simulink model "voertuig_cvs1"  (Simulink 8.0)
settings: Solver=ode45  StartTime=0.0  StopTime=simtijd  MaxStep=0.2  RelTol=1e-3
values from neighbouring files (symbols this model uses):
  Cw = 0.3    [voertuigmodel_rvv.m]
  fr = 0.014    [voertuigmodel_rvv.m]
  g = 9.81    [voertuigmodel_rvv.m]
  i = [1 2 3 4 5; 12 7.5 5.5 4.5 3.75]'    [voertuigmodel_rvv.m]
  J1 = 1.2    [voertuigmodel_rvv.m]
  J2 = 5.4    [voertuigmodel_rvv.m]
  m = 950    [voertuigmodel_rvv.m]
  mu_max = 1.05    [voertuigmodel_rvv.m]
  Nm_motor = [0 1000 2000 3000 4000 5000 6000 6500 7000; 50 90 90 95 100 90 85 80 0]'    [voertuigmodel_rvv.m]
  r = 0.3    [voertuigmodel_rvv.m]
  rho = 1.29    [voertuigmodel_rvv.m]
  v_i = [1 2 3 4 5;0 4.17 8.89 13.89 19.44]'    [voertuigmodel_rvv.m]
libraries: simulink x2
settings Model: Creator=879618  LastModifiedBy=879618
settings DataIOCC: SignalLoggingSaveFormat=ModelDataLogs
settings DebuggingCC: FcnCallInpInsideContextMsg=EnableAllAsWarning
settings GRTTargetCC: CombineOutputUpdateFcns=off  GRTInterface=on

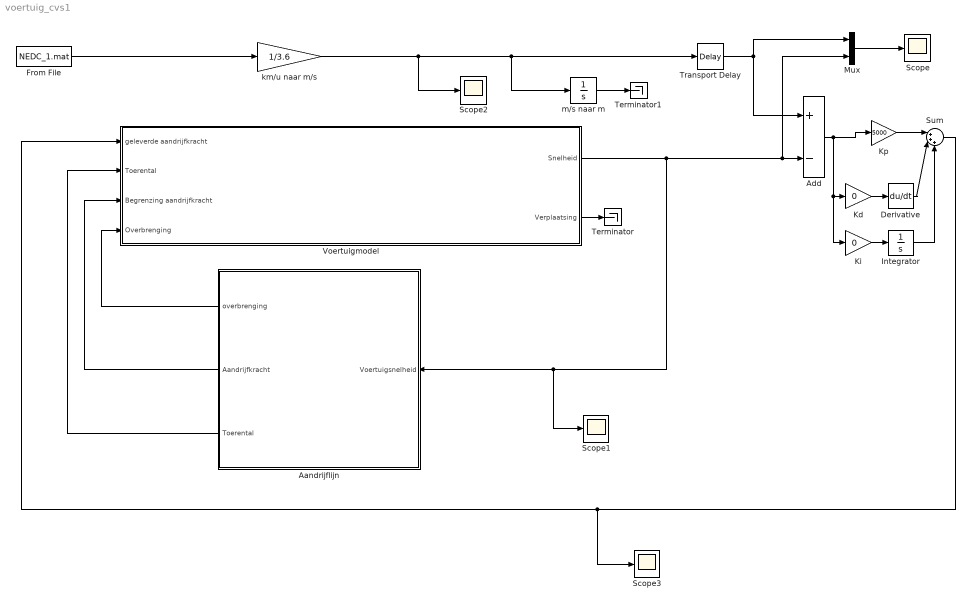
== system voertuig_cvs1 ==
  Aandrijflijn : Subsystem
  Add : Sum  Inputs=+-
  Derivative : Derivative
  From File : FromFile  FileName=NEDC_1.mat  SampleTime=1
  Integrator : Integrator
  Kd : Gain  Gain=0
  Ki : Gain  Gain=0
  Kp : Gain  Gain=5000
  Mux : Mux  Inputs=2
  Scope{,1..3} (4 alike) : Scope
      Scope settings: TimeRange=7.746100053792361  YMin=-2000  YMax=12000
      Scope1 settings: YMin=-2.5  YMax=35
      Scope2 settings: TimeRange=1200  YMin=6.037499999999994  YMax=6.737499999999997  SaveName=ScopeData5
      Scope3 settings: YMin=-2.5  YMax=35  SaveName=ScopeData3
  Sum : Sum  Inputs=|+++
  Terminator : Terminator
  Terminator1 : Terminator
  Transport Delay : TransportDelay  DelayTime=2
  Voertuigmodel : Subsystem
  km/u naar m/s : Gain  Gain=1/3.6
  m/s naar m : Integrator
  wires:
  Aandrijflijn/1(overbrenging) -> Voertuigmodel/4(Overbrenging)
  Aandrijflijn/3(Toerental) -> Voertuigmodel/2(Toerental)
  Aandrijflijn/2(Aandrijfkracht) -> Voertuigmodel/3(Begrenzing aandrijfkracht)
  Voertuigmodel/2(Verplaatsing) -> Terminator/1
  From File/1 -> km/u naar m/s/1
  Mux/1 -> Scope/1
  Add/1 -> Ki/1, Kd/1, Kp/1
  km/u naar m/s/1 -> m/s naar m/1, Transport Delay/1, Scope2/1
  Kp/1 -> Sum/1
  Kd/1 -> Derivative/1
  Sum/1 -> Scope3/1, Voertuigmodel/1(geleverde aandrijfkracht)
  Derivative/1 -> Sum/2
  m/s naar m/1 -> Terminator1/1
  Voertuigmodel/1(Snelheid) -> Mux/2, Add/2, Aandrijflijn/1(Voertuigsnelheid), Scope1/1
  Transport Delay/1 -> Add/1, Mux/1
  Ki/1 -> Integrator/1
  Integrator/1 -> Sum/3

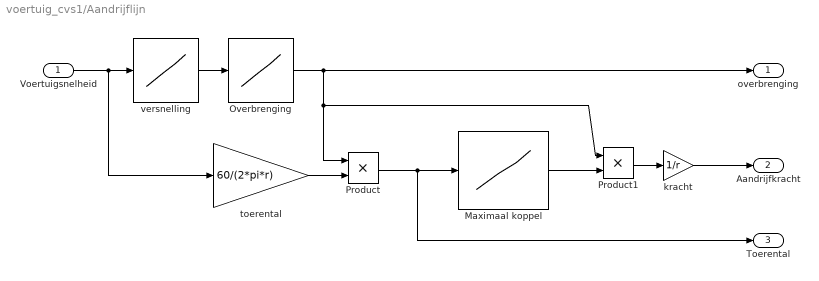
== system voertuig_cvs1/Aandrijflijn ==
  Voertuigsnelheid : Inport
  Maximaal koppel : Lookup_n-D  NumberOfTableDimensions=1  BreakpointsForDimension1=Nm_motor(:,1)  Table=Nm_motor(:,2)  RndMeth=Simplest  InputSameDT=on
  Overbrenging : Lookup_n-D  NumberOfTableDimensions=1  BreakpointsForDimension1=[1:5]  Table=i(:,2)  InterpMethod=Flat  RndMeth=Simplest  InputSameDT=on
  Product : Product  RndMeth=Zero
  Product1 : Product  RndMeth=Zero
  kracht : Gain  Gain=1/r
  toerental : Gain  Gain=60/(2*pi*r)
  versnelling : Lookup_n-D  NumberOfTableDimensions=1  BreakpointsForDimension1=v_i(:,2)  Table=v_i(:,1)  InterpMethod=Flat  RndMeth=Simplest  InputSameDT=on
  overbrenging : Outport
  Aandrijfkracht : Outport  Port=2
  Toerental : Outport  Port=3
  wires:
  versnelling/1 -> Overbrenging/1
  Overbrenging/1 -> overbrenging/1, Product/1, Product1/1
  Voertuigsnelheid/1 -> versnelling/1, toerental/1
  Maximaal koppel/1 -> Product1/2
  Product1/1 -> kracht/1
  kracht/1 -> Aandrijfkracht/1
  Product/1 -> Toerental/1, Maximaal koppel/1
  toerental/1 -> Product/2

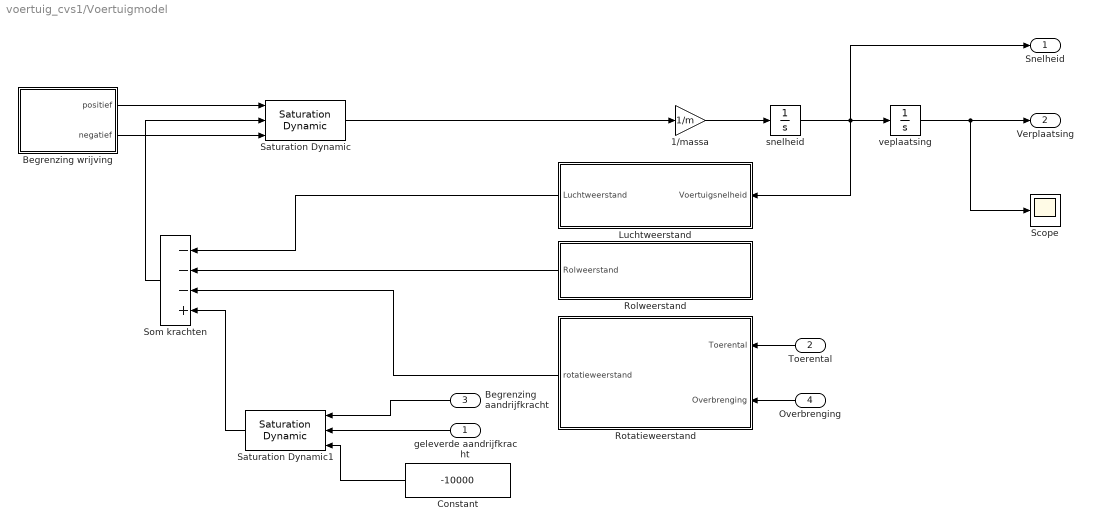
== system voertuig_cvs1/Voertuigmodel ==
  geleverde aandrijfkracht : Inport
  Toerental : Inport  Port=2
  Begrenzing aandrijfkracht : Inport  Port=3
  Overbrenging : Inport  Port=4
  1/massa : Gain  Gain=1/m
  Begrenzing wrijving : Subsystem
  Constant : Constant  Value=-10000
  Luchtweerstand : Subsystem
  Rolweerstand : Subsystem
  Rotatieweerstand : Subsystem
  Saturation Dynamic : simulink/Discontinuities/Saturation Dynamic  OutMin=[]  OutMax=[]  OutDataTypeStr=Inherit: Same as second input  OutDataType=fixdt(1, 16)  OutScaling=2^-10  DoSatur=off
  Saturation Dynamic1 : simulink/Discontinuities/Saturation Dynamic  OutMin=[]  OutMax=[]  OutDataTypeStr=Inherit: Same as second input  OutDataType=fixdt(1, 16)  OutScaling=2^-10  DoSatur=off
  Scope : Scope
      settings: TimeRange=3.873050026896181  YMin=-518.6403508771944  YMax=878.2894736842086  SaveName=ScopeData2
  Som krachten : Sum  Inputs=---+
  snelheid : Integrator
  veplaatsing : Integrator
  Snelheid : Outport
  Verplaatsing : Outport  Port=2
  wires:
  1/massa/1 -> snelheid/1
  snelheid/1 -> veplaatsing/1, Luchtweerstand/1(Voertuigsnelheid), Snelheid/1
  veplaatsing/1 -> Verplaatsing/1, Scope/1
  Saturation Dynamic/1 -> 1/massa/1
  Begrenzing aandrijfkracht/1 -> Saturation Dynamic1/1
  geleverde aandrijfkracht/1 -> Saturation Dynamic1/2
  Saturation Dynamic1/1 -> Som krachten/4
  Som krachten/1 -> Saturation Dynamic/2
  Luchtweerstand/1(Luchtweerstand) -> Som krachten/1
  Rolweerstand/1(Rolweerstand) -> Som krachten/2
  Begrenzing wrijving/1(positief) -> Saturation Dynamic/1
  Toerental/1 -> Rotatieweerstand/1(Toerental)
  Overbrenging/1 -> Rotatieweerstand/2(Overbrenging)
  Begrenzing wrijving/2(negatief) -> Saturation Dynamic/3
  Constant/1 -> Saturation Dynamic1/3
  Rotatieweerstand/1(rotatieweerstand) -> Som krachten/3

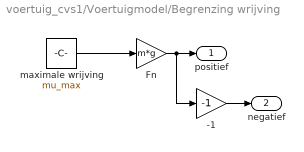
== system voertuig_cvs1/Voertuigmodel/Begrenzing wrijving ==
  -1 : Gain  Gain=-1
  Fn : Gain  Gain=m*g
  maximale wrijving : Constant  Value=mu_max
  positief : Outport
  negatief : Outport  Port=2
  wires:
  maximale wrijving/1 -> Fn/1
  Fn/1 -> -1/1, positief/1
  -1/1 -> negatief/1

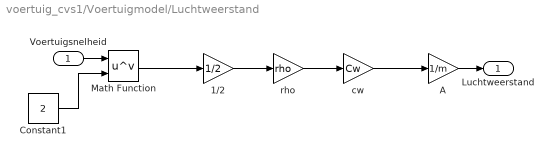
== system voertuig_cvs1/Voertuigmodel/Luchtweerstand ==
  Voertuigsnelheid : Inport
  1/2 : Gain  Gain=1/2
  A : Gain  Gain=1/m
  Constant1 : Constant  Value=2
  Math Function : Math  Operator=pow  SaturateOnIntegerOverflow=on
  cw : Gain  Gain=Cw
  rho : Gain  Gain=rho
  Luchtweerstand : Outport
  wires:
  1/2/1 -> rho/1
  rho/1 -> cw/1
  cw/1 -> A/1
  Math Function/1 -> 1/2/1
  Constant1/1 -> Math Function/2
  Voertuigsnelheid/1 -> Math Function/1
  A/1 -> Luchtweerstand/1

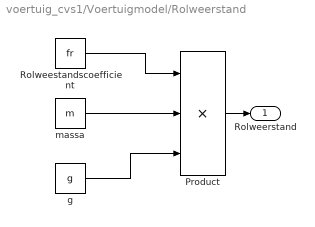
== system voertuig_cvs1/Voertuigmodel/Rolweerstand ==
  Product : Product  Inputs=3  RndMeth=Zero
  Rolweestandscoefficient : Constant  Value=fr
  g : Constant  Value=g
  massa : Constant  Value=m
  Rolweerstand : Outport
  wires:
  Rolweestandscoefficient/1 -> Product/1
  massa/1 -> Product/2
  g/1 -> Product/3
  Product/1 -> Rolweerstand/1

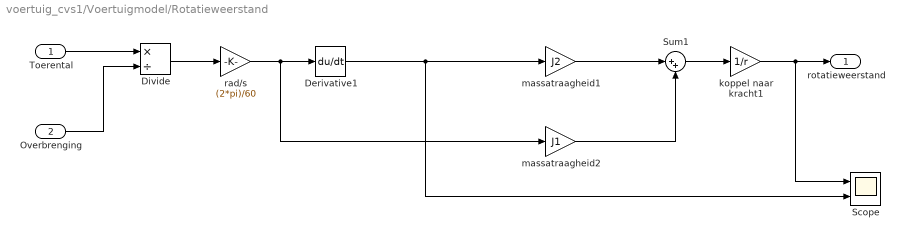
== system voertuig_cvs1/Voertuigmodel/Rotatieweerstand ==
  Toerental : Inport
  Overbrenging : Inport  Port=2
  Derivative1 : Derivative
  Divide : Product  Inputs=*/
  Scope : Scope  NumInputPorts=2
      settings: YMin=-5~-5  YMax=5~5  SaveName=ScopeData4
  Sum1 : Sum  Inputs=|++
  koppel naar kracht1 : Gain  Gain=1/r
  massatraagheid1 : Gain  Gain=J2
  massatraagheid2 : Gain  Gain=J1
  rad/s : Gain  Gain=(2*pi)/60
  rotatieweerstand : Outport
  wires:
  rad/s/1 -> Derivative1/1, massatraagheid2/1
  Derivative1/1 -> massatraagheid1/1, Scope/2
  massatraagheid1/1 -> Sum1/1
  massatraagheid2/1 -> Sum1/2
  Sum1/1 -> koppel naar kracht1/1
  koppel naar kracht1/1 -> rotatieweerstand/1, Scope/1
  Overbrenging/1 -> Divide/2
  Toerental/1 -> Divide/1
  Divide/1 -> rad/s/1
